simulink model "Node_NM"  (R2024b)
settings: Solver=ode1  StartTime=0.0  StopTime=10.0  FixedStep=0.5e-3  RelTol=1e-3
settings Model: Creator=wai484  LastModifiedBy=wai484
settings SolverCC: EnableFixedStepZeroCrossing=on
settings DataIOCC: SaveOutput=off  SaveTime=off
settings ModelReferenceCC: ModelReferenceMinAlgLoopOccurrences=on
settings GRTTargetCC: CombineOutputUpdateFcns=off

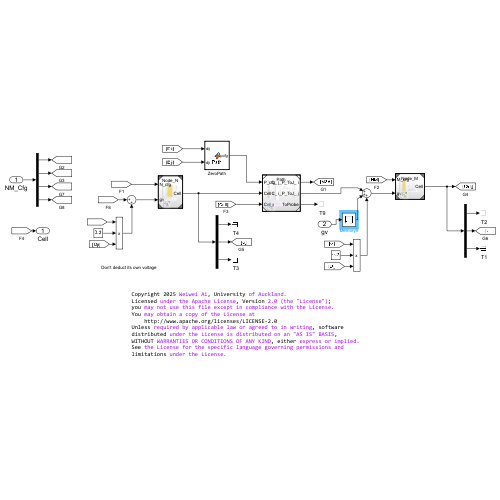
[thumbnail: Simulink's stored preview of the top-level diagram]
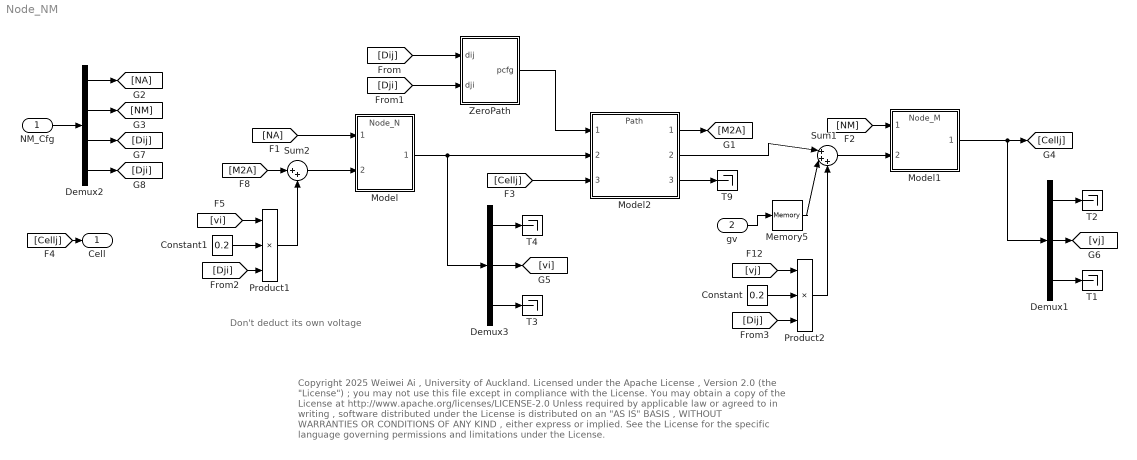
== system Node_NM ==
  note: Don't deduct its own voltage
  note: Copyright 2025 Weiwei Ai , University of Auckland.
      | Licensed under the Apache License , Version 2.0 (the "License") ;
      | you may not use this file except in compliance with the License.
      | You may obtain a copy of the License at
      | http://www.apache.org/licenses/LICENSE-2.0
      | Unless required by applicable law or agreed to in writing , software
      | distributed under the License is distributed on an "AS IS" BASIS ,
      | WITHOUT WARRANTIES OR CONDITIONS OF ANY KIND , either express or implied.
      | See the License for the specific language governing permissions and
      | limitations under the License.
  NM_Cfg : Inport  OutDataTypeStr=double  PortDimensions=52
  gv : Inport  Port=2  OutDataTypeStr=double  PortDimensions=1
  Constant : Constant  Value=0.2
  Constant1 : Constant  Value=0.2
  Demux1 : Demux  Outputs=[1,1,4]
  Demux2 : Demux  Outputs=[24,26,1,1]
  Demux3 : Demux  Outputs=[1,1,4]
  Memory5 : Memory  InheritSampleTime=on  LinearizeMemory=on  LinearizeAsDelay=on
  Model : ModelReference  ModelNameDialog=Node_N.slx  SimulationMode=Normal  ModelReferenceVersion=1.15
  Model1 : ModelReference  ModelNameDialog=Node_M.slx  SimulationMode=Normal  ModelReferenceVersion=1.8
  Model2 : ModelReference  ModelNameDialog=Path.slx  SimulationMode=Normal  ModelReferenceVersion=1.7
  Product1 : Product  Inputs=***
  Product2 : Product  Inputs=***
  Sum1 : Sum  Inputs=|+++
  Sum2 : Sum  Inputs=|++
  T{1..4,9} (5 alike) : Terminator
  ZeroPath : MATLAB Function  TreatAsAtomicUnit=on
  Cell : Outport  OutDataTypeStr=double  PortDimensions=6  SampleTime=0
  wires:
  NM_Cfg/1 -> Demux2/1
  Model2/3 -> T9/1
  Demux2/1 -> [NA]
  Demux2/2 -> [NM]
  [NA] -> Model/1
  [NM] -> Model1/1
  Model2/1 -> [M2A]
  Model1/1 -> [Cellj], Demux1/1
  [Cellj] -> Model2/3
  [Cellj] -> Cell/1
  ZeroPath/1(pcfg) -> Model2/1
  Model2/2 -> Sum1/1
  Sum1/1 -> Model1/2
  Demux1/3 -> T1/1
  Demux1/1 -> T2/1
  Model/1 -> Demux3/1, Model2/2
  Demux3/3 -> T3/1
  Demux3/1 -> T4/1
  Demux3/2 -> [vi]
  Demux1/2 -> [vj]
  Constant/1 -> Product2/2
  [vj] -> Product2/1
  Product2/1 -> Sum1/3
  [M2A] -> Sum2/1
  Sum2/1 -> Model/2
  Constant1/1 -> Product1/2
  [vi] -> Product1/1
  Product1/1 -> Sum2/2
  Demux2/3 -> [Dij]
  Demux2/4 -> [Dji]
  [Dij] -> ZeroPath/1(dij)
  [Dji] -> ZeroPath/2(dji)
  [Dji] -> Product1/3
  [Dij] -> Product2/3
  Memory5/1 -> Sum1/2
  gv/1 -> Memory5/1

== matlab function Node_NM/ZeroPath ==
  data: pcfg output; dij input; dji input
function pcfg= Path(dij,dji)
%#codegen
CVi2j=1;
Dij=dij;
aij=1;
bij=0;
cij=0;

CVj2i=1;
Dji=dji;
aji=1;
bji=0;
cji=0;
C=5;

pcfg=[CVi2j,Dij, aij, bij, cij,CVj2i,Dji, aji,bji,cji,C];
end
